simulink model "traj_optim_integral"  (R2024b)
settings: Solver=VariableStepAuto  StartTime=0.0  StopTime=30  RelTol=1e-3
model workspace (MAT data in the model file):
  controller_type : ControllerType (value not decoded)
  dtime = 0.04
  g = 9.8
  max_iter = 400
  steps = 400
  vehicle = Vehicle
  vehicle.m = 100000
  vehicle.L = 30
  vehicle.I = 30000000
  vehicle.Len = 60
  vehicle.max_gimbal = 0.174532925199
  vehicle.min_thrust = 440000
  vehicle.max_thrust = 2210000
  vehicle.Name = "Astra2"
  x0 = [0 1000 0 -80 0 0]
values from neighbouring files (symbols this model uses):
  vehicle = Vehicle(100000,30,60,deg2rad(20),800000,2000000, Name = "Default")    [CasADi_MPC.m]
undefined symbols (not defined in the file or in its folder): F, Light, MIL
libraries: simulink_extras x3, aerolibanim x1, sharedTrackingLibrary x1, aerolibwind2 x1
settings Model: SimulationMode=accelerator  Creator=alexa  LastModifiedBy=thatf

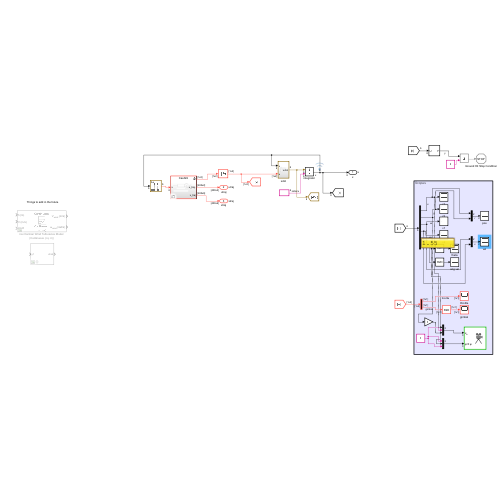
[thumbnail: Simulink's stored preview of the top-level diagram]
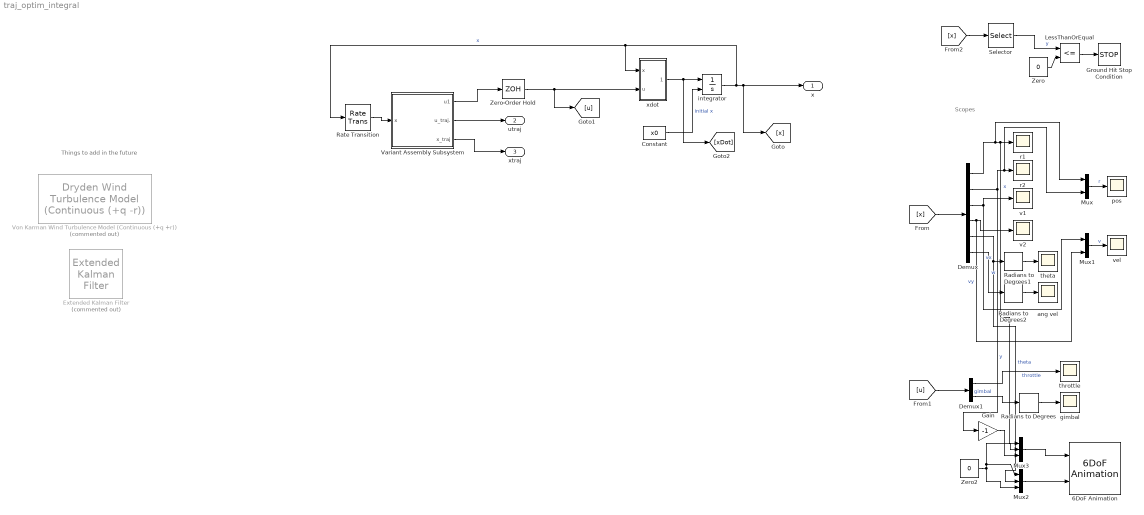
== system traj_optim_integral ==
  note: Scopes
  note: Things to add in the future
  6DoF Animation : aerolibanim/6DoF Animation  u1=[-10 10 -1 1 0 10]  u2=0.1  u3=1.0  u4=[0, 0, 0]  u5=Fly alongside  u6=[0,8,0]  u7=40  u8=on
  Constant : Constant  Value=x0
  Demux : Demux  Outputs=6
  Demux1 : Demux  Outputs=2
  Extended Kalman Filter : sharedTrackingLibrary/Extended Kalman Filter  Commented=on  StateTransitionFcn=myStateTransitionFcn  HasStateTransitionJacobianFcn=off  HasAdditiveProcessNoise=Additive  ProcessNoise=1  HasTimeVaryingProcessNoise=off  HasStateTransitionFcnExtraArgument=0  InitialState=0  InitialStateCovariance=1  MeasurementFcn1=myMeasurementFcn  HasMeasurementJacobianFcn1=off  HasMeasurementEnablePort1=off  HasAdditiveMeasurementNoise1=Additive  MeasurementNoise1=1  HasTimeVaryingMeasurementNoise1=off  HasMeasurementFcnExtraArgument1=0  HasMeasurementWrapping1=off  MeasurementFcn2=myMeasurementFcn  HasMeasurementJacobianFcn2=off  HasMeasurementEnablePort2=off  HasAdditiveMeasurementNoise2=Additive  MeasurementNoise2=1  HasTimeVaryingMeasurementNoise2=off  HasMeasurementFcnExtraArgument2=0  HasMeasurementWrapping2=off  MeasurementFcn3=myMeasurementFcn  HasMeasurementJacobianFcn3=off  HasMeasurementEnablePort3=off  HasAdditiveMeasurementNoise3=Additive  MeasurementNoise3=1  HasTimeVaryingMeasurementNoise3=off  HasMeasurementFcnExtraArgument3=0  HasMeasurementWrapping3=off  MeasurementFcn4=myMeasurementFcn  HasMeasurementJacobianFcn4=off  HasMeasurementEnablePort4=off  HasAdditiveMeasurementNoise4=Additive  MeasurementNoise4=1  HasTimeVaryingMeasurementNoise4=off  HasMeasurementFcnExtraArgument4=0  HasMeasurementWrapping4=off  MeasurementFcn5=myMeasurementFcn  HasMeasurementJacobianFcn5=off  HasMeasurementEnablePort5=off  HasAdditiveMeasurementNoise5=Additive  MeasurementNoise5=1  HasTimeVaryingMeasurementNoise5=off  HasMeasurementFcnExtraArgument5=0  HasMeasurementWrapping5=off  EnableMultirate=off  StateTransitionFcnSampleTime=1  MeasurementFcn1SampleTime=1  MeasurementFcn2SampleTime=1  MeasurementFcn3SampleTime=1  MeasurementFcn4SampleTime=1  MeasurementFcn5SampleTime=1  UseCurrentEstimator=on  OutputStateCovariance=off  DataType=double  SampleTime=1  NumberOfMeasurements=1
  Gain : Gain  Gain=-1
  Ground Hit Stop Condition : Stop
  LessThanOrEqual : RelationalOperator  Operator=<=  OutDataTypeStr=boolean  RndMeth=Simplest  InputSameDT=off
  Mux : Mux  Inputs=2
  Mux1 : Mux  Inputs=2
  Mux2 : Mux  Inputs=3
  Mux3 : Mux  Inputs=3
  Radians to Degrees : simulink_extras/Transformations/Radians to Degrees
  Radians to Degrees1 : simulink_extras/Transformations/Radians to Degrees
  Radians to Degrees2 : simulink_extras/Transformations/Radians to Degrees
  Rate Transition : RateTransition  OutPortSampleTime=dtime
  Selector : Selector  InputPortWidth=6  IndexOptions=Index vector (dialog)  Indices=[2]  OutputSizes=1
  Variant Assembly Subsystem : Subsystem  Variant=on  VariantChoicesSpecifier={}  VariantChoicesEnumeration=ControllerType  VariantControlVariable=controller_type
  Von Karman Wind Turbulence Model (Continuous (+q +r)) : aerolibwind2/Dryden Wind Turbulence Model  (Continuous (+q -r))  Commented=on  units=Metric (MKS)  spec=MIL-F-8785C  model=Continuous Von Karman (+q +r)  W20=15  Wdeg=0  TurbProb=10^-2 - Light  L_high=762  Wingspan=10  ts=0.1  Seed=[23341 23342 23343 23344]  T_on=on
      settings: LibrarySourceBlock=|
      | aerolibwind2/Von Karman Wind Turbulence Model
      | (Continuous (+q +r))
  Zero : Constant  Value=0  OutDataTypeStr=Inherit: Inherit via back propagation
  Zero-Order Hold : ZeroOrderHold  SampleTime=-1
  Zero2 : Constant  Value=0  OutDataTypeStr=Inherit: Inherit via back propagation
  ang vel : Scope
  gimbal : Scope
  integrator : Integrator  InitialConditionSource=external
  pos : Scope
  r1 : Scope
  r2 : Scope
  theta : Scope
  throttle : Scope
  v1 : Scope
  v2 : Scope
  vel : Scope
  xdot : Subsystem
  x : Outport  SignalName=x
  utraj : Outport  Port=2  SignalName=utraj
  xtraj : Outport  Port=3  SignalName=xtraj
  wires:
  Constant/1 -> integrator/2  "initial x"
  xdot/1(x dot) -> [xDot], integrator/1
  integrator/1 -> [x], x/1, Rate Transition/1, xdot/1(x)  "x"
  Rate Transition/1 -> Variant Assembly Subsystem/1(x)
  Variant Assembly Subsystem/3(x_traj) -> xtraj/1
  Variant Assembly Subsystem/1(u1) -> Zero-Order Hold/1
  Zero-Order Hold/1 -> [u], xdot/2(u)
  Mux/1 -> pos/1  "r"
  Demux/6 -> Radians to Degrees2/1  "w"
  Demux/3 -> v1/1, Mux1/1  "vx"
  Demux/2 -> Mux/2, r2/1, Gain/1  "y"
  Demux/5 -> Mux2/2, Radians to Degrees1/1  "theta"
  Demux/1 -> Mux/1, Mux3/1, r1/1  "x"
  Mux1/1 -> vel/1  "v"
  Demux/4 -> Mux1/2, v2/1  "vy"
  [x] -> Demux/1
  [u] -> Demux1/1
  Demux1/1 -> throttle/1  "throttle"
  Demux1/2 -> Radians to Degrees/1  "gimbal"
  Radians to Degrees/1 -> gimbal/1
  LessThanOrEqual/1 -> Ground Hit Stop Condition/1
  Zero/1 -> LessThanOrEqual/2
  [x] -> Selector/1
  Selector/1 -> LessThanOrEqual/1  "y"
  Radians to Degrees1/1 -> theta/1
  Radians to Degrees2/1 -> ang vel/1
  Variant Assembly Subsystem/2(u_traj.) -> utraj/1
  Mux2/1 -> 6DoF Animation/2
  Mux3/1 -> 6DoF Animation/1
  Zero2/1 -> Mux2/1, Mux3/2, Mux2/3
  Gain/1 -> Mux3/3

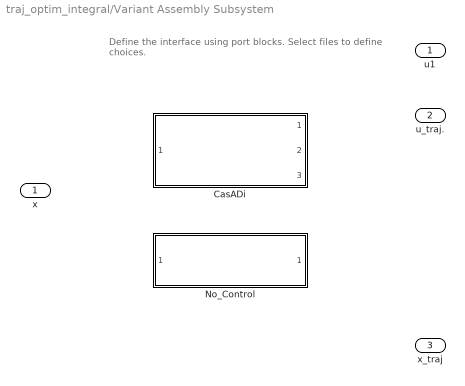
== system traj_optim_integral/Variant Assembly Subsystem ==
  note: Define the interface using port blocks.
      | Select files to define choices.
  x : Inport
  CasADi : Subsystem  VariantControl=controller_type == ControllerType.CasADi  ReferencedSubsystem=CasADi
  No_Control : Subsystem  VariantControl=controller_type == ControllerType.No_Control  ReferencedSubsystem=No_Control
  u1 : Outport
  u_traj. : Outport  Port=2
  x_traj : Outport  Port=3

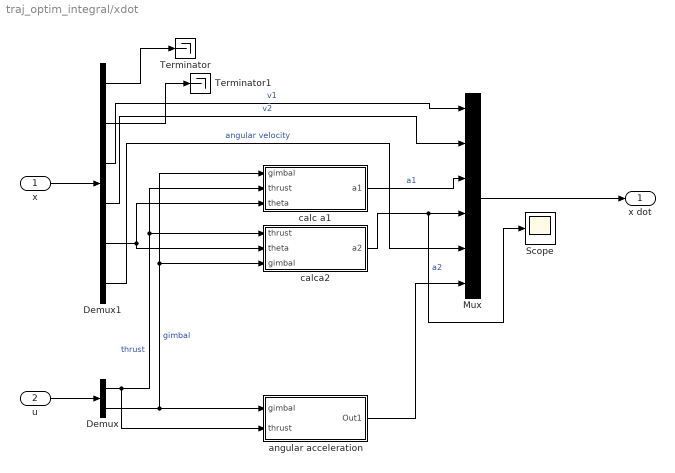
== system traj_optim_integral/xdot ==
  x : Inport
  u : Inport  Port=2
  Demux : Demux  Outputs=2
  Demux1 : Demux  Outputs=6
  Mux : Mux  Inputs=6
  Scope : Scope
  Terminator : Terminator
  Terminator1 : Terminator
  angular acceleration : Subsystem
  calc a1 : Subsystem
  calca2 : Subsystem
  x dot : Outport
  wires:
  Mux/1 -> x dot/1
  u/1 -> Demux/1
  x/1 -> Demux1/1
  Demux1/3 -> Mux/1  "v1"
  Demux1/4 -> Mux/2  "v2"
  Demux1/6 -> Mux/5  "angular velocity"
  Demux1/5 -> calca2/2(theta), calc a1/3(theta)
  Demux/1 -> angular acceleration/2(thrust), calc a1/2(thrust), calca2/1(thrust)  "thrust"
  Demux/2 -> angular acceleration/1(gimbal), calc a1/1(gimbal), calca2/3(gimbal)  "gimbal"
  calc a1/1(a1) -> Mux/3  "a1"
  calca2/1(a2) -> Scope/1, Mux/4  "a2"
  angular acceleration/1(Out1) -> Mux/6
  Demux1/1 -> Terminator/1
  Demux1/2 -> Terminator1/1

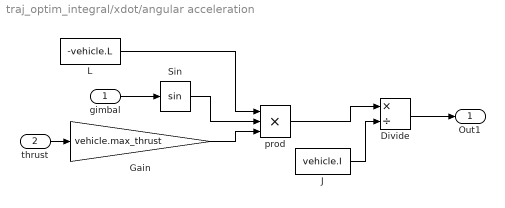
== system traj_optim_integral/xdot/angular acceleration ==
  gimbal : Inport
  thrust : Inport  Port=2
  Divide : Product  Inputs=*/
  Gain : Gain  Gain=vehicle.max_thrust
  J : Constant  Value=vehicle.I
  L : Constant  Value=-vehicle.L
  Sin : Trigonometry
  prod : Product  Inputs=3
  Out1 : Outport
  wires:
  prod/1 -> Divide/1
  gimbal/1 -> Sin/1
  Sin/1 -> prod/2
  L/1 -> prod/1
  J/1 -> Divide/2
  Divide/1 -> Out1/1
  thrust/1 -> Gain/1
  Gain/1 -> prod/3

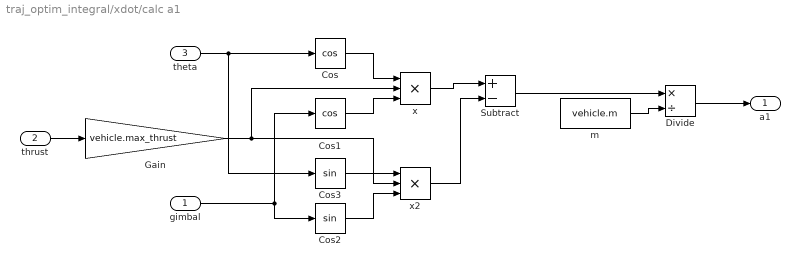
== system traj_optim_integral/xdot/calc a1 ==
  gimbal : Inport
  thrust : Inport  Port=2
  theta : Inport  Port=3
  Cos : Trigonometry  Operator=cos
  Cos1 : Trigonometry  Operator=cos
  Cos2 : Trigonometry
  Cos3 : Trigonometry
  Divide : Product  Inputs=*/
  Gain : Gain  Gain=vehicle.max_thrust
  Subtract : Sum  Inputs=+-
  m : Constant  Value=vehicle.m
  x : Product  Inputs=3
  x2 : Product  Inputs=3
  a1 : Outport
  wires:
  gimbal/1 -> Cos1/1, Cos2/1
  theta/1 -> Cos3/1, Cos/1
  Cos/1 -> x/1
  Cos1/1 -> x/3
  x/1 -> Subtract/1
  m/1 -> Divide/2
  Divide/1 -> a1/1
  x2/1 -> Subtract/2
  Subtract/1 -> Divide/1
  Cos3/1 -> x2/1
  Cos2/1 -> x2/3
  thrust/1 -> Gain/1
  Gain/1 -> x2/2, x/2

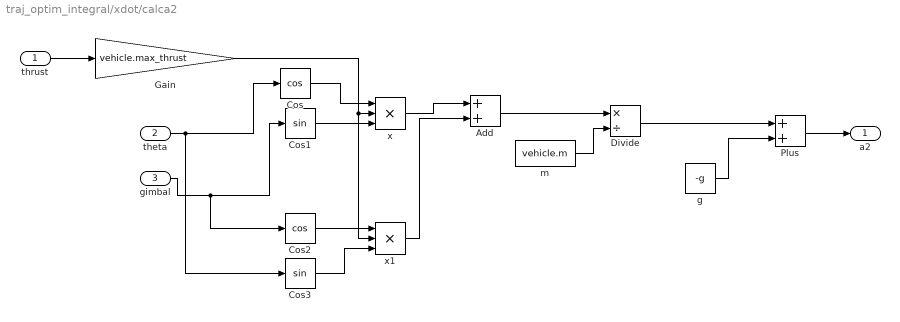
== system traj_optim_integral/xdot/calca2 ==
  thrust : Inport
  theta : Inport  Port=2
  gimbal : Inport  Port=3
  Add : Sum
  Cos : Trigonometry  Operator=cos
  Cos1 : Trigonometry
  Cos2 : Trigonometry  Operator=cos
  Cos3 : Trigonometry
  Divide : Product  Inputs=*/
  Gain : Gain  Gain=vehicle.max_thrust
  Plus : Sum
  g : Constant  Value=-g
  m : Constant  Value=vehicle.m
  x : Product  Inputs=3
  x1 : Product  Inputs=3
  a2 : Outport
  wires:
  x/1 -> Add/1
  Cos/1 -> x/1
  Cos1/1 -> x/3
  m/1 -> Divide/2
  Divide/1 -> Plus/1
  Add/1 -> Divide/1
  g/1 -> Plus/2
  Plus/1 -> a2/1
  Cos3/1 -> x1/3
  Cos2/1 -> x1/1
  thrust/1 -> Gain/1
  theta/1 -> Cos/1, Cos3/1
  gimbal/1 -> Cos2/1, Cos1/1
  Gain/1 -> x/2, x1/2
  x1/1 -> Add/2
